simulink model "observer"  (R2020b)
settings: Solver=VariableStepAuto  StartTime=0.0  StopTime=10.0  RelTol=1e-3
values from neighbouring files (symbols this model uses):
  A = eval(nA0)    [Linearization.m]    (also in calib_up_up.m)
  B = eval(nB0)    [Linearization.m]    (also in calib_up_up.m)
  C = [0 0 1 0 0 ... (first row only)    [Linearization.m]    (also in calib_up_up.m)
  L = place(A', C', po).'    [calib_up_up.m]    (also in tune_parameters.m = 500)
  obs_x0 = [0;0;0;0;0]    [calib_up_up.m]
settings Model: Creator=cmatteo  LastModifiedBy=llaporte

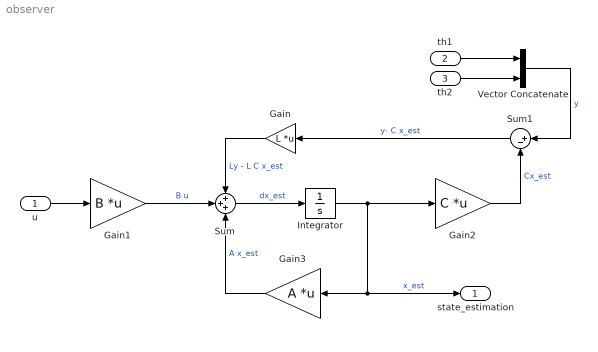
== system observer ==
  u : Inport
  th1 : Inport  Port=2
  th2 : Inport  Port=3
  Gain : Gain  Gain=L  Multiplication=Matrix(K*u)
  Gain1 : Gain  Gain=B  Multiplication=Matrix(K*u)
  Gain2 : Gain  Gain=C  Multiplication=Matrix(K*u)
  Gain3 : Gain  Gain=A  Multiplication=Matrix(K*u)
  Integrator : Integrator  InitialCondition=obs_x0
  Sum : Sum  Inputs=+++
  Sum1 : Sum  Inputs=|+-
  Vector Concatenate : Concatenate
  state_estimation : Outport
  wires:
  u/1 -> Gain1/1
  Gain1/1 -> Sum/2  "B u"
  Sum/1 -> Integrator/1  "dx_est"
  Integrator/1 -> Gain2/1, state_estimation/1, Gain3/1  "x_est"
  Gain2/1 -> Sum1/2  "Cx_est"
  Sum1/1 -> Gain/1  "y- C x_est"
  Gain3/1 -> Sum/3  "A x_est"
  Gain/1 -> Sum/1  "Ly - L C x_est"
  th2/1 -> Vector Concatenate/2
  th1/1 -> Vector Concatenate/1
  Vector Concatenate/1 -> Sum1/1  "y"
